simulink model "Sim_02"  (R2025b)
settings: Solver=ode4  StartTime=0.0  StopTime=10.0  FixedStep=0.01  RelTol=1e-3
undefined symbols (not defined in the file or in its folder): Ga, Kd, Kp
settings Model: Creator=diegoalfonsocosta  LastModifiedBy=diegoalfonsocosta

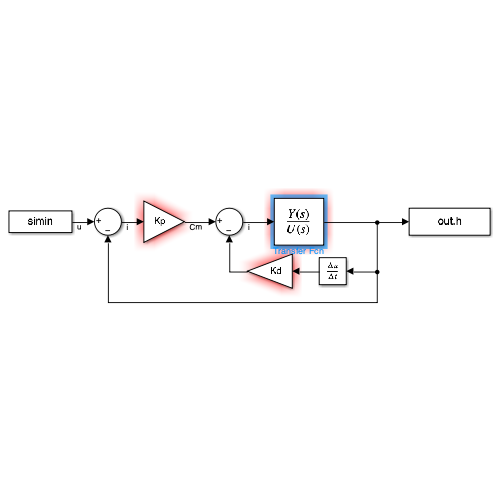
[thumbnail: Simulink's stored preview of the top-level diagram]
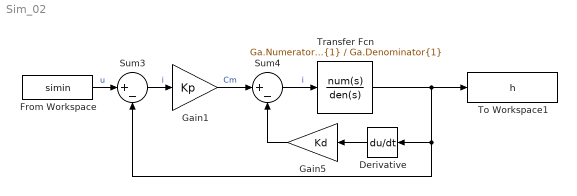
== system Sim_02 ==
  Derivative : Derivative
  From Workspace : FromWorkspace  VariableName=simin
  Gain1 : Gain  Gain=Kp
  Gain5 : Gain  Gain=Kd
  Sum3 : Sum  Inputs=|+-
  Sum4 : Sum  Inputs=|+-
  To Workspace1 : ToWorkspace  VariableName=h  SaveFormat=Timeseries  SampleTime=-1
  Transfer Fcn : TransferFcn  Numerator=Ga.Numerator{1}  Denominator=Ga.Denominator{1}
  wires:
  From Workspace/1 -> Sum3/1  "u"
  Sum3/1 -> Gain1/1  "i"
  Gain1/1 -> Sum4/1  "Cm"
  Sum4/1 -> Transfer Fcn/1  "i"
  Derivative/1 -> Gain5/1
  Gain5/1 -> Sum4/2
  Transfer Fcn/1 -> To Workspace1/1, Derivative/1, Sum3/2
